simulink model "system_model"  (R2024a)
settings: Solver=VariableStepAuto  StartTime=0.0  StopTime=100000.0  MaxStep=1  RelTol=1e-9
values from neighbouring files (symbols this model uses):
  a_leader = 500*10^3 + earth_radi    (= 6871000)    [main.m]    (also in main_2.m)
  B_f_max = (C_d*A_f_max)/m_f    (= 0.78)    [main_2.m]
  B_f_min = (C_d*A_f_min)/m_f    (= 0.13)    [main_2.m]
  B_l_max = (C_d*A_l_max)/m_l    (= 0.78)    [main_2.m]
  B_l_min = (C_d*A_l_min)/m_l    (= 0.13)    [main_2.m]
  earth_radi = 6371*10^3    (= 6371000)    [main.m]    (also in main_2.m)
  J = eye(3)    [attitude.m]    (also in state_func.m = 43943563035.8; state_func_test.m = J_2 * R_E^2)
  J_2 = 1.08263 * 10^(-3)    (= 0.00108263)    [main.m]    (also in main_2.m; state_func.m)
  Kd = 5    [attitude.m]
  Kp = 5    [attitude.m]
  m_f = 1    [main.m]    (also in main_2.m = 2)
  m_l = 1    [main.m]    (also in main_2.m = 2)
  mu = 13/ 26.98    (= 0.481838398814)    [drag_coefficent_ruff_estimation.m]    (also in main.m = 6.67e-11; main_2.m = 398589196000000; state_func.m = 398589196000000; untitled5.m)
  q_0 = q_0 /norm(q_0)    [attitude.m]
  rho_leader = mean_rho_500km    (= 7.3e-13)    [main_2.m]
  w_0 = [1; 2; 1]    [attitude.m]
  x = theta_vec    [drag_coefficent_ruff_estimation.m]    (also in main.m = [d_a; d_lambda; d_e_x; d_e_y; d_i_x; d_i_y; d_Ballistic]; main_2.m = [d_a; d_lambda; d_e_x; d_e_y; d_i_x; d_i_y])
  x_f_prop = [a_follower; m_follower; e_follower; omega_follower; Omega_follower; i_follower]    [main_2.m]
  x_l_prop = [a_leader; m_leader; e_leader; omega_leader; Omega_leader; i_leader]    [main_2.m]
libraries: mpclib x1, slpidlib x1
(part 1 of 2)
settings Model: Creator=andrefan  LastModifiedBy=andre
settings DataIOCC: FinalStateName=system_modelSimState  InitialState=system_modelSimState  SaveFinalState=on  SaveOperatingPoint=on
settings RTWCC: GPUComputeCapability=3.5

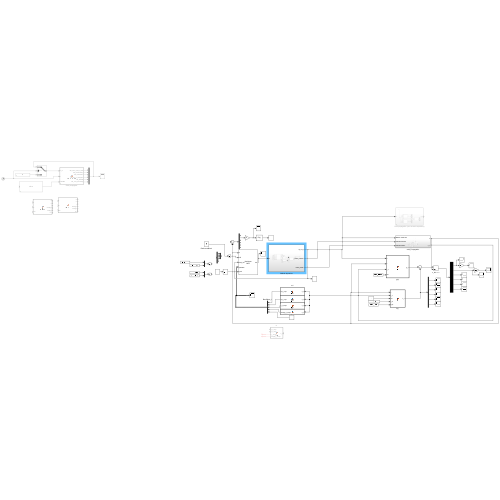
[thumbnail: Simulink's stored preview of the top-level diagram]
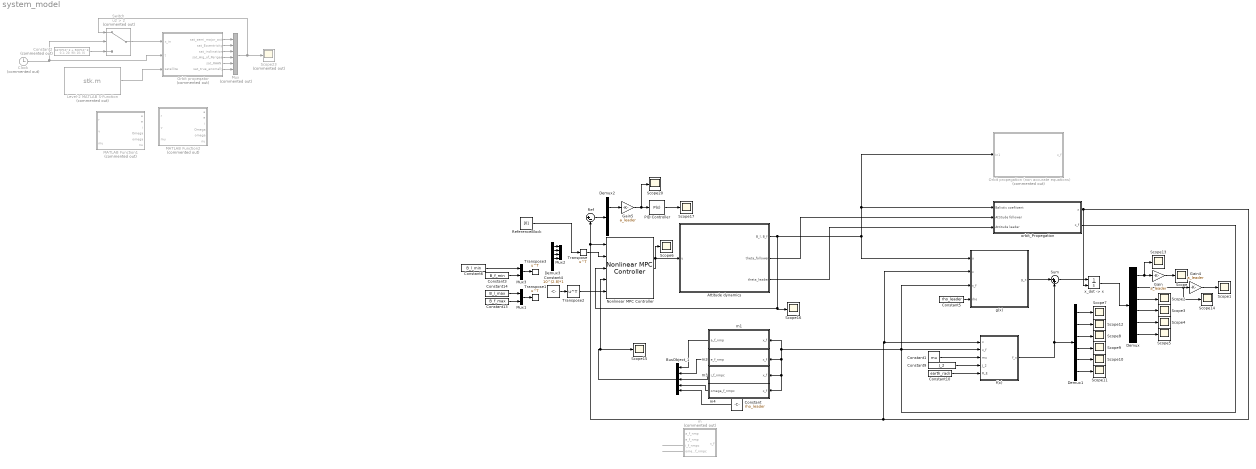
== system system_model ==
  Attitude dynamics : Subsystem
  BusObject_1 : BusCreator  Inputs=5  OutDataTypeStr=Bus: BusObject  NonVirtualBus=on
      settings: InheritFromInputs=off
  Clock : Clock  Commented=on
  Constant : Constant  Value=rho_leader
  Constant1 : Constant  Value=mu
  Constant10 : Constant  Value=earth_radi
  Constant13 : Constant  Value=B_f_max
  Constant14 : Constant  Value=B_l_max
  Constant2 : Constant  Commented=on  Value=|
      | [6370*10^3 + 500*10^3; 0.1;
      | 20; 90;
      | 10;
      | 0]
  Constant3 : Constant  Value=B_f_min
  Constant4 : Constant  Value=10^(2.8)*1
  Constant5 : Constant  Value=rho_leader
  Constant6 : Constant  Value=B_l_min
  Constant9 : Constant  Value=J_2
  Demux{,1..3} (4 alike) : Demux  Outputs=6
  Gain : Gain  Gain=a_leader
  Gain4 : Gain  Gain=a_leader
  Gain5 : Gain  Gain=a_leader
  Level-2 MATLAB S-Function : M-S-Function  Commented=on  FunctionName=stk.m
  MATLAB Function1 : MATLAB Function  Commented=on  TreatAsAtomicUnit=on
  MATLAB Function2 : MATLAB Function  Commented=on  TreatAsAtomicUnit=on
  Mux : Mux  Commented=on  Inputs=6
  Mux1 : Mux  Inputs=2
  Mux2 : Mux
  Mux3 : Mux  Inputs=2
  Nonlinear MPC Controller : mpclib/Nonlinear MPC Controller  nlmpcobj=nlobj  UseObjectTs=on  TsControl=20  UseMEX=off  md_enabled=off  mvtarget_enabled=off  param_enabled=on  cost_enabled=off  mvseq_enabled=off  stateseq_enabled=off  ovseq_enabled=off  slack_enabled=off  status_enabled=off  ov_min=off  ov_max=off  mv_min=off  mv_max=off  mvrate_min=off  mvrate_max=off  state_min=off  state_max=off  ov_weight=on  mv_weight=off  mvrate_weight=off  ecr_weight=off  nlp_initialize=off
  Orbit propegation (non accurate equations) : Subsystem  Commented=on
  Orbit propegator : MATLAB Function  Commented=on  TreatAsAtomicUnit=on
  PID Controller : slpidlib/PID Controller  Controller=P  Form=Parallel  TimeDomain=Continuous-time  UseExternalTs=off  SampleTime=-1  IntegratorMethod=Forward Euler  FilterMethod=Forward Euler  ControllerParametersSource=internal  P=500  I=0.002  UseKiTs=off  D=0  UseExternalDerivativeSource=off  N=100  UseFilter=on  TunerSelectOption=Transfer Function Based (PID Tuner App)  InitialConditionSource=internal  InitialConditionForIntegrator=0  InitialConditionForFilter=0  DifferentiatorICPrevScaledInput=0  ExternalReset=none  TrackingMode=off  Kt=1  LimitOutput=off  SatLimitsSource=internal  UpperSaturationLimit=inf  LowerSaturationLimit=-inf  LinearizeAsGain=on  AntiWindupMode=none  Kb=1  LimitIntegrator=off  UpperIntegratorSaturationLimit=inf  LowerIntegratorSaturationLimit=-inf  POutMin=[]  POutMax=[]  IOutMin=[]  IOutMax=[]  DOutMin=[]  DOutMax=[]  NOutMin=[]  NOutMax=[]  SumOutMin=[]  SumOutMax=[]  SaturationOutMin=[]  SaturationOutMax=[]  PParamMin=[]  PParamMax=[]  IParamMin=[]  IParamMax=[]  DParamMin=[]  DParamMax=[]  NParamMin=[]  NParamMax=[]  KbParamMin=[]  KbParamMax=[]  KtParamMin=[]  KtParamMax=[]  KbOutMin=[]  KbOutMax=[]  KtOutMin=[]  KtOutMax=[]  IntegratorOutMin=[]  IntegratorOutMax=[]  FilterOutMin=[]  FilterOutMax=[]  SumI1OutMin=[]  SumI1OutMax=[]  SumI2OutMin=[]  SumI2OutMax=[]  SumI3OutMin=[]  SumI3OutMax=[]  SumI4OutMin=[]  SumI4OutMax=[]  SumDOutMin=[]  SumDOutMax=[]  DifferentiatorOutMin=[]  DifferentiatorOutMax=[]  FilterDiffOutCoefMin=[]  FilterDiffOutCoefMax=[]  ReciprocalOutMin=[]  ReciprocalOutMax=[]  SumDenOutMin=[]  SumDenOutMax=[]  SumNumOutMin=[]  SumNumOutMax=[]  DivideOutMin=[]  DivideOutMax=[]  UdiffTsProdOutMin=[]  UdiffTsProdOutMax=[]  NTsProdOutMin=[]  NTsProdOutMax=[]  UintegralTsProdOutMin=[]  UintegralTsProdOutMax=[]  UngainTsProdOutMin=[]  UngainTsProdOutMax=[]  ClampingZeroOutDataTypeStr=Inherit: Inherit via back propagation  ClampingZeroOutMin=[]  ClampingZeroOutMax=[]  FilterDenConstantOutDataTypeStr=Inherit: Inherit via back propagation  FilterDenConstantOutMin=[]  FilterDenConstantOutMax=[]  PCopyOutDataTypeStr=Inherit: Inherit via back propagation  PCopyOutMin=[]  PCopyOutMax=[]  NCopyOutDataTypeStr=Inherit: Inherit via back propagation  NCopyOutMin=[]  NCopyOutMax=[]  IntegratorContinuousStateAttributes=''  IntegratorStateMustResolveToSignalObject=off  IntegratorRTWStateStorageClass=Auto  FilterContinuousStateAttributes=''  FilterStateMustResolveToSignalObject=off  FilterRTWStateStorageClass=Auto  ParallelPVariant=InternalParameters  IdealPVariant=Disabled  IVariant=Disabled  DVariant=Disabled  IntegratorVariant=Disabled  SatVariant=Disabled  AWVariant=Disabled  PCopyVariant=Disabled  TRVariant=Disabled  FdbkBlocksVariant=Forward  IdealPFdbkVariant=Disabled  SatFdbkVariant=Disabled  DerivativeFilterVariant=Disabled  NVariant=Disabled  NCopyVariant=Disabled_SignalSpec  FilterICVariant=Disabled  IntegratorICVariant=Disabled  ExternalResetVariant=Disabled  TRSumVariant=Passthrough  SumFdbkVariant=Disabled  SumVariant=Passthrough_P  TsampFilterVariant=InternalTs  TsampNgainVariant=Passthrough  TsampIntegralVariant=Disabled_SignalSpec  ExternalSaturationOutDataTypeStr=Inherit: Same as second input  DerivativeSourceVariant=Disabled
  Ref : Sum  Inputs=|+-
  ReferenceBlock : Constant  Value=[0]
  Scope{,1..17,20} (19 alike) : Scope
  Scope23 : Scope  Commented=on
  Sum : Sum  Inputs=|++
  Switch : Switch  Commented=on  Criteria=u2 > Threshold  Threshold=2  SaturateOnIntegerOverflow=off  InputSameDT=off
  Transpose{,1..3} (4 alike) : Math  Operator=transpose
  f(x) : MATLAB Function  TreatAsAtomicUnit=on
  g(x) : MATLAB Function  TreatAsAtomicUnit=on
  m : MATLAB Function  Commented=on  TreatAsAtomicUnit=on
  m1 : MATLAB Function  TreatAsAtomicUnit=on
  m2 : MATLAB Function  TreatAsAtomicUnit=on
  m3 : MATLAB Function  TreatAsAtomicUnit=on
  m4 : MATLAB Function  TreatAsAtomicUnit=on
  orbit_Propegation : Subsystem
  "x_dot -> x" : Integrator  InitialConditionSource=external  InitialCondition=x
  wires:
  g(x)/1(g_x) -> Sum/1
  Sum/1 -> "x_dot -> x"/1
  "x_dot -> x"/1 -> Demux/1
  f(x)/1(f_x) -> Demux1/1, Sum/2
  Constant1/1 -> f(x)/3(mu)
  Constant5/1 -> g(x)/4(rho)
  Constant9/1 -> f(x)/4(J_2)
  Constant10/1 -> f(x)/5(R_E)
  Demux/3 -> Scope2/1
  Demux/2 -> Scope14/1, Gain4/1
  Demux/1 -> Scope13/1, Gain/1
  Demux/5 -> Scope4/1
  Demux/6 -> Scope5/1
  Demux/4 -> Scope3/1
  Gain/1 -> Scope/1
  Demux1/2 -> Scope12/1
  Gain4/1 -> Scope1/1
  Ref/1 -> Demux2/1
  PID Controller/1 -> Scope17/1
  Demux2/2 -> Gain5/1
  Gain5/1 -> PID Controller/1, Scope20/1
  Attitude dynamics/1("B_l, B_f") -> Scope16/1, Nonlinear MPC Controller/3, g(x)/1(u), Orbit propegation (non accurate equations)/1(In1), orbit_Propegation/1(Balistic coefiicent)
  Clock/1 -> Orbit propegator/2(t), Switch/2
  Constant2/1 -> Switch/3
  Switch/1 -> Orbit propegator/1(x_in)
  Orbit propegator/1(sat_semi_major_axis) -> Mux/1
  Orbit propegator/2(sat_Eccentricity) -> Mux/2
  Orbit propegator/3(sat_inclination) -> Mux/3
  Orbit propegator/4(sat_Arg_of_Perigee) -> Mux/4
  Orbit propegator/5(sat_RAAN) -> Mux/5
  Orbit propegator/6(sat_true_anomally) -> Mux/6
  Mux/1 -> Scope23/1, Switch/1
  Level-2 MATLAB S-Function/1 -> Orbit propegator/3(satellite)
  Attitude dynamics/3(theta_leader) -> orbit_Propegation/3(Attitude leader)
  Attitude dynamics/2(theta_follower) -> orbit_Propegation/2(Attitude follower)
  Nonlinear MPC Controller/1 -> Scope6/1, Attitude dynamics/1(u)
  Constant14/1 -> Mux1/1
  Constant13/1 -> Mux1/2
  Mux1/1 -> Transpose1/1
  Demux1/1 -> Scope7/1
  Demux1/3 -> Scope8/1
  Demux1/4 -> Scope9/1
  Demux1/5 -> Scope10/1
  Demux1/6 -> Scope11/1
  orbit_Propegation/2(x_f) -> m4/1(x_f), m3/1(x_f), m2/1(x_f), m1/1(x_f), f(x)/2(x_f), g(x)/3(x_f)
  BusObject_1/1 -> Scope15/1, Nonlinear MPC Controller/4
  ReferenceBlock/1 -> Transpose/1
  Demux3/1 -> Mux2/1
  Demux3/2 -> Mux2/2
  Demux3/3 -> Mux2/3
  Demux3/4 -> Mux2/4
  orbit_Propegation/1(x) -> "x_dot -> x"/2, g(x)/2(x), f(x)/1(x), Ref/2, Nonlinear MPC Controller/1
  Transpose/1 -> Nonlinear MPC Controller/2
  Constant/1 -> BusObject_1/5
  m/4(omega_f_nmpc) -> ?
  m/3(i_f_nmpc) -> ?
  m1/1(a_f_nmp) -> BusObject_1/1
  m2/1(e_f_nmp) -> BusObject_1/2
  m3/1(i_f_nmpc) -> BusObject_1/3
  m4/1(omega_f_nmpc) -> BusObject_1/4
  Constant4/1 -> Transpose2/1
  Transpose2/1 -> Nonlinear MPC Controller/5
  Constant3/1 -> Mux3/2
  Constant6/1 -> Mux3/1
  Mux3/1 -> Transpose3/1

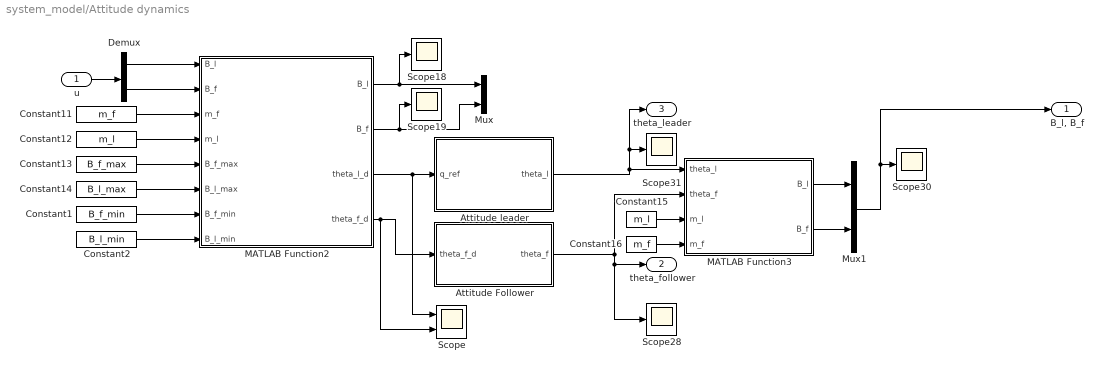
== system system_model/Attitude dynamics ==
  u : Inport
  Attitude Follower : Subsystem
  Attitude leader : Subsystem
  Constant1 : Constant  Value=B_f_min
  Constant11 : Constant  Value=m_f
  Constant12 : Constant  Value=m_l
  Constant13 : Constant  Value=B_f_max
  Constant14 : Constant  Value=B_l_max
  Constant15 : Constant  Value=m_l
  Constant16 : Constant  Value=m_f
  Constant2 : Constant  Value=B_l_min
  Demux : Demux  Outputs=2
  MATLAB Function2 : MATLAB Function  TreatAsAtomicUnit=on
  MATLAB Function3 : MATLAB Function  TreatAsAtomicUnit=on
  Mux : Mux  Inputs=2
  Mux1 : Mux  Inputs=2
  Scope : Scope  NumInputPorts=2
  Scope{18..19,28,30..31} (5 alike) : Scope
  "B_l, B_f" : Outport
  theta_follower : Outport  Port=2
  theta_leader : Outport  Port=3
  wires:
  Constant11/1 -> MATLAB Function2/3(m_f)
  Attitude leader/1(theta_l) -> theta_leader/1, Scope31/1, MATLAB Function3/1(theta_l)
  MATLAB Function2/1(B_l) -> Scope18/1, Mux/1
  Attitude Follower/1(theta_f) -> theta_follower/1, Scope28/1, MATLAB Function3/2(theta_f)
  Demux/2 -> MATLAB Function2/2("B_f ")
  Constant12/1 -> MATLAB Function2/4(m_l)
  MATLAB Function3/1(B_l) -> Mux1/1
  MATLAB Function2/2(B_f) -> Scope19/1, Mux/2
  Constant13/1 -> MATLAB Function2/5(B_f_max)
  Constant14/1 -> MATLAB Function2/6(B_l_max)
  MATLAB Function2/4(theta_f_d) -> Scope/2, Attitude Follower/1(theta_f_d)
  MATLAB Function3/2(B_f) -> Mux1/2
  MATLAB Function2/3(theta_l_d) -> Scope/1, Attitude leader/1(q_ref)
  Constant16/1 -> MATLAB Function3/4(m_f)
  Constant15/1 -> MATLAB Function3/3(m_l)
  Mux1/1 -> "B_l, B_f"/1, Scope30/1
  Constant1/1 -> MATLAB Function2/7(B_f_min)
  Constant2/1 -> MATLAB Function2/8(B_l_min)
  u/1 -> Demux/1
  Demux/1 -> MATLAB Function2/1("B_l ")

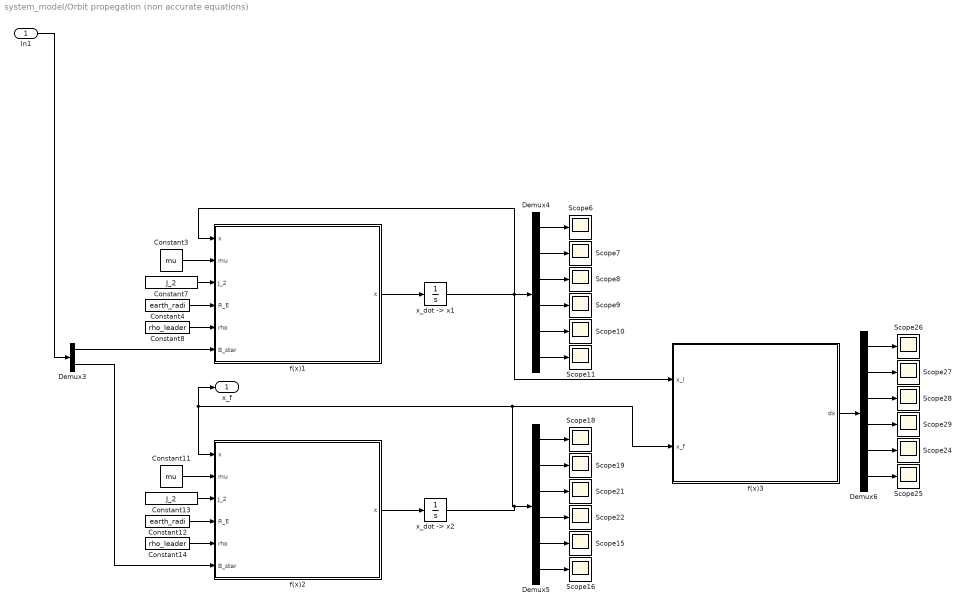
== system system_model/Orbit propegation (non accurate equations) ==
  In1 : Inport
  Constant11 : Constant  Value=mu
  Constant12 : Constant  Value=earth_radi
  Constant13 : Constant  Value=J_2
  Constant14 : Constant  Value=rho_leader
  Constant3 : Constant  Value=mu
  Constant4 : Constant  Value=earth_radi
  Constant7 : Constant  Value=J_2
  Constant8 : Constant  Value=rho_leader
  Demux3 : Demux  Outputs=2
  Demux4 : Demux  Outputs=6
  Demux5 : Demux  Outputs=6
  Demux6 : Demux  Outputs=6
  Scope{6..11,15..16,18..19,21..22,24..29} (18 alike) : Scope
  f(x)1 : MATLAB Function  TreatAsAtomicUnit=on
  f(x)2 : MATLAB Function  TreatAsAtomicUnit=on
  f(x)3 : MATLAB Function  TreatAsAtomicUnit=on
  "x_dot -> x1" : Integrator  InitialCondition=x_l_prop
  "x_dot -> x2" : Integrator  InitialCondition=x_f_prop
  x_f : Outport
  wires:
  Demux4/6 -> Scope11/1
  Constant4/1 -> f(x)1/4(R_E)
  Constant7/1 -> f(x)1/3(J_2)
  Demux3/2 -> f(x)2/6(B_star)
  Demux4/5 -> Scope10/1
  Constant8/1 -> f(x)1/5(rho)
  Demux4/4 -> Scope9/1
  Demux5/4 -> Scope22/1
  Demux5/2 -> Scope19/1
  Demux6/4 -> Scope29/1
  Demux3/1 -> f(x)1/6(B_star)
  Demux4/2 -> Scope7/1
  Constant14/1 -> f(x)2/5(rho)
  Demux4/3 -> Scope8/1
  Constant12/1 -> f(x)2/4(R_E)
  Demux5/5 -> Scope15/1
  Constant11/1 -> f(x)2/2(mu)
  "x_dot -> x1"/1 -> f(x)1/1("x "), Demux4/1, f(x)3/1(x_l)
  Demux5/6 -> Scope16/1
  Demux6/5 -> Scope24/1
  "x_dot -> x2"/1 -> Demux5/1, f(x)3/2(x_f), x_f/1, f(x)2/1("x ")
  Demux6/1 -> Scope26/1
  Demux6/3 -> Scope28/1
  Demux5/1 -> Scope18/1
  f(x)2/1(x) -> "x_dot -> x2"/1
  Constant13/1 -> f(x)2/3(J_2)
  Demux6/2 -> Scope27/1
  Constant3/1 -> f(x)1/2(mu)
  Demux5/3 -> Scope21/1
  Demux6/6 -> Scope25/1
  Demux4/1 -> Scope6/1
  f(x)3/1(dx) -> Demux6/1
  f(x)1/1(x) -> "x_dot -> x1"/1
  In1/1 -> Demux3/1

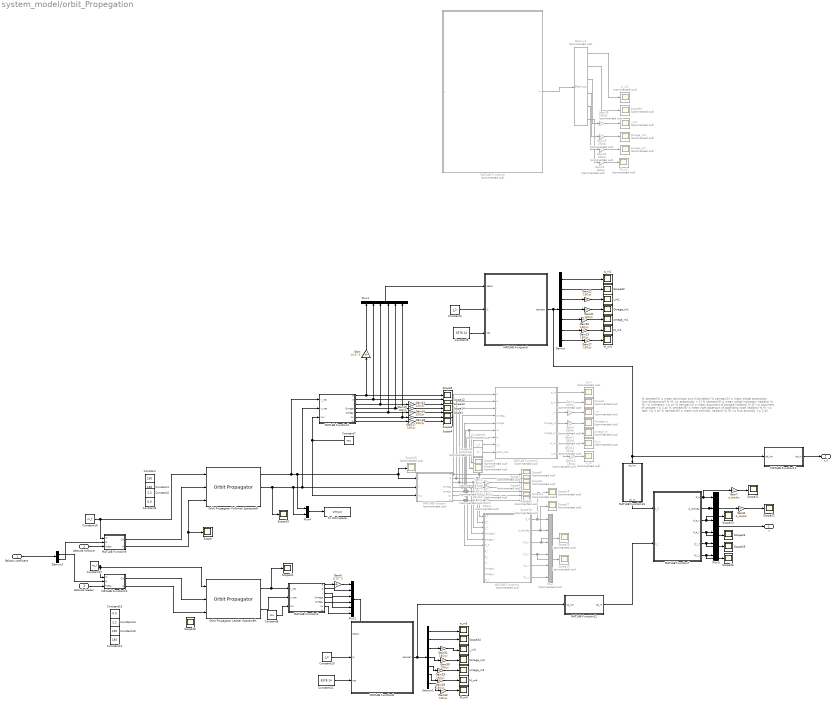
== system system_model/orbit_Propegation ==
  note: % oemean(1) = mean semimajor axis (kilometers)
      | % oemean(2) = mean orbital eccentricity (non-dimensional)
      | % (0 <= eccentricity < 1)
      | % oemean(3) = mean orbital inclination (radians)
      | % (0 <= inclination <= pi)
      | % oemean(4) = mean argument of perigee (radians)
      | % (0 <= argument of perigee <= 2 pi)
      | % oemean(5) = mean right ascension of ascending node (radians)
      | % (0 <= raan <= 2 pi)
      | % oemean(6) = mean true anomaly (radians)
      | % (0 <= true anomaly <= 2 pi)
  Balistic coefiicent : Inport
  Attitude follower : Inport  Port=2
  Attitude leader : Inport  Port=3
  Constant{,1,12..13} (4 alike) : Constant  Value=150
  Constant10 : Constant  Value=J_2
  Constant11 : Constant  Value=6378.14
  Constant14 : Constant  Value=2.2
  Constant15 : Constant  Value=0.0
  Constant16 : Constant  Value=m_f
  Constant17 : Constant  Value=m_l
  Constant2 : Constant  Value=2.2
  Constant3 : Constant  Value=J_2
  Constant4 : Constant  Value=0.0
  Constant5 : Constant  Commented=on  Value=J_2
  Constant6 : Constant  Commented=on  Value=earth_radi
  Constant7 : Constant  Value=mu
  Constant8 : Constant  Value=mu
  Constant9 : Constant  Value=6378.14
  Demux : Demux  Outputs=7
  Demux1 : Demux  Commented=on  Outputs=6
  Demux2 : Demux  Outputs=7
  Demux3 : Demux  Outputs=2
  Gain : Gain  Gain=1/10^3
  Gain{1..5,9..13,23..26} (14 alike) : Gain  Commented=on  Gain=180/pi
  Gain{14..22,27..32} (15 alike) : Gain  Gain=180/pi
  Gain6 : Gain  Gain=1/10^3
  Gain7 : Gain  Gain=a_leader
  Gain8 : Gain  Gain=a_leader
  MATLAB Function : MATLAB Function  Commented=on  TreatAsAtomicUnit=on
  MATLAB Function1 : MATLAB Function  Commented=on  TreatAsAtomicUnit=on
  MATLAB Function10 : MATLAB Function  TreatAsAtomicUnit=on
  MATLAB Function11 : MATLAB Function  TreatAsAtomicUnit=on
  MATLAB Function12 : MATLAB Function  TreatAsAtomicUnit=on
  MATLAB Function13 : MATLAB Function  TreatAsAtomicUnit=on
  MATLAB Function2 : MATLAB Function  TreatAsAtomicUnit=on
  MATLAB Function3 : MATLAB Function  TreatAsAtomicUnit=on
  MATLAB Function4 : MATLAB Function  Commented=on  TreatAsAtomicUnit=on
  MATLAB Function5 : MATLAB Function  TreatAsAtomicUnit=on
  MATLAB Function6 : MATLAB Function  Commented=on  TreatAsAtomicUnit=on
  MATLAB Function7 : MATLAB Function  TreatAsAtomicUnit=on
  MATLAB Function8 : MATLAB Function  TreatAsAtomicUnit=on
  MATLAB Function9 : MATLAB Function  TreatAsAtomicUnit=on
  M_m : Scope  Commented=on
  M_m{1,3..5} (4 alike) : Scope
  M_m2 : Scope  Commented=on
  Mux : Mux  Commented=on  Inputs=6
  Mux1 : Mux  Inputs=6
  Mux2 : Mux  Inputs=6
  Mux3 : Mux  Inputs=6
  Mux4 : Mux  Inputs=2
  Omega_m : Scope  Commented=on
  Omega_m1 : Scope
  Omega_m2 : Scope  Commented=on
  Omega_m3 : Scope
  Orbit Propagator Follower Spacecraft : OrbitPropagator  propagator=Numerical (high precision)  dateOut=off  massSrc=Port  mass=2.0  inclination=20  argPeriapsis=25  trueAnomaly=100  inertialPosition=[3649700.0 3308200.0 -4676600.0]  inertialVelocity=[-2750.8 6666.4 2573.4]  fixedPosition=[-4142689.0 -2676864.7 -4669861.6]  fixedVelocity=[1452.7 -6720.7 2568.1]  gravityModel=Oblate ellipsoid (J2)  customR=3396200  customMu=4.305e13  customJ2=1.0826269e-03  customOmega=4.06125949e-3  outputTransform=on  useDrag=on  useOxygen=off  dragCoeffSrc=Port  dragCoeff=2.3  dragAreaSrc=Port  dragArea=0.6
  Orbit Propagator Leader Spacecraft : OrbitPropagator  propagator=Numerical (high precision)  dateOut=off  massSrc=Port  mass=2.0  inclination=20  argPeriapsis=25  trueAnomaly=100.001  inertialPosition=[3649700.0 3308200.0 -4676600.0]  inertialVelocity=[-2750.8 6666.4 2573.4]  fixedPosition=[-4142689.0 -2676864.7 -4669861.6]  fixedVelocity=[1452.7 -6720.7 2568.1]  gravityModel=Oblate ellipsoid (J2)  customR=3396200  customMu=4.305e13  customJ2=1.0826269e-03  customOmega=4.06125949e-3  useDrag=on  useOxygen=off  dragCoeffSrc=Port  dragCoeff=2.3  dragAreaSrc=Port  dragArea=0.6
  Scope{,1,3..5,12..14,16,21..26,30..32,34} (19 alike) : Scope
  Scope{2,6..11,15,17..20,27..29,33} (16 alike) : Scope  Commented=on
  To Workspace : ToWorkspace  VariableName=simout  SaveFormat=Timeseries  SampleTime=-1
  a_m : Scope  Commented=on
  a_m1 : Scope
  a_m2 : Scope  Commented=on
  a_m3 : Scope
  i_m : Scope  Commented=on
  i_m1 : Scope
  i_m2 : Scope  Commented=on
  i_m3 : Scope
  omega_m : Scope  Commented=on
  omega_m1 : Scope
  omega_m2 : Scope  Commented=on
  omega_m3 : Scope
  u_m : Scope  Commented=on
  x : Outport
  x_f : Outport  Port=2
  wires:
  MATLAB Function/1(a) -> MATLAB Function4/1(a_f), Scope6/1, MATLAB Function1/1(a)
  MATLAB Function4/4(d_e_y) -> Scope29/1, Mux/4
  Gain9/1 -> Scope10/1
  Orbit Propagator Follower Spacecraft/1 -> Mux4/1, MATLAB Function/1(r), Scope15/1, MATLAB Function2/1(r_vec)
  Orbit Propagator Leader Spacecraft/1 -> MATLAB Function3/1(r_vec), Scope31/1
  MATLAB Function4/1(d_a) -> Scope19/1, Mux/1
  MATLAB Function4/6(d_i_y) -> Mux/6
  Gain3/1 -> Scope9/1
  MATLAB Function/3(i) -> MATLAB Function4/3(i_f), Gain1/1, MATLAB Function1/3(i)
  MATLAB Function/7(M) -> MATLAB Function4/6(M_f), Gain10/1, Scope17/1, MATLAB Function1/7(M)
  MATLAB Function4/5(d_i_x) -> Mux/5
  Gain1/1 -> Scope8/1
  Constant7/1 -> MATLAB Function/3(mu), MATLAB Function2/3(mu)
  MATLAB Function/6(nu) -> Gain2/1, Scope20/1, MATLAB Function1/6(nu)
  MATLAB Function4/3(d_e_x) -> Scope28/1, Mux/3
  MATLAB Function4/2(d_lambda) -> Scope27/1, Mux/2
  Gain2/1 -> Scope11/1
  MATLAB Function/2(e) -> MATLAB Function4/2(e_f), Scope7/1, MATLAB Function1/2(e)
  Constant8/1 -> MATLAB Function3/3(mu)
  Gain10/1 -> Scope18/1
  MATLAB Function1/1(a_m) -> a_m/1
  Constant5/1 -> MATLAB Function1/8(J_2)
  Constant6/1 -> MATLAB Function1/9(earth_radi)
  MATLAB Function1/2(e_m) -> Scope2/1
  MATLAB Function1/3(i_m) -> Gain4/1
  MATLAB Function1/4(Omega_m) -> Gain5/1
  MATLAB Function1/5(omega_m) -> Gain11/1
  MATLAB Function1/6(M_m) -> Gain12/1
  Gain4/1 -> i_m/1
  Gain5/1 -> Omega_m/1
  Gain11/1 -> omega_m/1
  Gain12/1 -> M_m/1
  MATLAB Function/5(omega) -> MATLAB Function1/5(omega), MATLAB Function4/5(omega_f), Gain9/1
  MATLAB Function/4(Omega) -> MATLAB Function1/4(Omega), MATLAB Function4/4(Omega_f), Gain3/1
  MATLAB Function1/7(u_m) -> Gain13/1
  Gain13/1 -> u_m/1
  Orbit Propagator Follower Spacecraft/2 -> Mux4/2, MATLAB Function/2(v), MATLAB Function2/2(v_vec), Scope16/1
  MATLAB Function2/7(M) -> Gain18/1
  MATLAB Function2/4(Omega) -> Gain15/1, Mux1/5
  MATLAB Function2/2(e) -> Scope12/1, Mux1/2
  MATLAB Function2/3(i) -> Gain14/1, Mux1/3
  MATLAB Function2/5(omega) -> Gain16/1, Mux1/4
  Gain14/1 -> Scope13/1
  Gain15/1 -> Scope14/1
  Gain16/1 -> Scope1/1
  Gain17/1 -> Scope3/1
  Gain18/1 -> Scope4/1
  Constant3/1 -> MATLAB Function5/2(j2)
  Constant9/1 -> MATLAB Function5/3(req)
  MATLAB Function2/1(a) -> Scope5/1, Gain/1
  MATLAB Function2/6(nu) -> Gain17/1, Mux1/6
  Gain/1 -> Mux1/1
  MATLAB Function5/1(oemean) -> Demux/1, MATLAB Function13/1(ob_km), MATLAB Function11/1(ob_km)
  Demux/6 -> Gain19/1
  Demux/3 -> Gain22/1
  Demux/5 -> Gain20/1
  Demux/2 -> Scope32/1
  Demux/1 -> a_m1/1
  Demux/4 -> Gain21/1
  Gain19/1 -> M_m1/1
  Gain20/1 -> omega_m1/1
  Gain21/1 -> Omega_m1/1
  Gain22/1 -> i_m1/1
  Demux1/2 -> Scope33/1
  Gain23/1 -> M_m2/1
  Gain25/1 -> Omega_m2/1
  Gain24/1 -> omega_m2/1
  Demux1/3 -> Gain26/1
  Gain26/1 -> i_m2/1
  Demux1/5 -> Gain24/1
  Demux1/4 -> Gain25/1
  Demux1/6 -> Gain23/1
  Demux1/1 -> a_m2/1
  MATLAB Function6/1(xn) -> Demux1/1
  Demux/7 -> Gain27/1
  Gain27/1 -> M_m3/1
  Mux1/1 -> MATLAB Function5/1(oeosc)
  Orbit Propagator Leader Spacecraft/2 -> MATLAB Function3/2(v_vec)
  MATLAB Function3/1(a) -> Gain6/1
  MATLAB Function3/2(e) -> Mux2/2
  MATLAB Function3/3(i) -> Mux2/3
  MATLAB Function3/6(nu) -> Mux2/6
  Demux2/7 -> Gain32/1
  Demux2/2 -> Scope34/1
  Demux2/5 -> Gain29/1
  Constant10/1 -> MATLAB Function8/2(j2)
  Gain30/1 -> Omega_m3/1
  Gain29/1 -> omega_m3/1
  Demux2/3 -> Gain31/1
  Gain31/1 -> i_m3/1
  Demux2/4 -> Gain30/1
  Demux2/6 -> Gain28/1
  Constant11/1 -> MATLAB Function8/3(req)
  Gain32/1 -> M_m5/1
  Gain28/1 -> M_m4/1
  Demux2/1 -> a_m3/1
  Mux2/1 -> MATLAB Function8/1(oeosc)
  MATLAB Function8/1(oemean) -> MATLAB Function12/1(ob_km), Demux2/1
  MATLAB Function7/6(d_i_y) -> Scope26/1, Mux3/6
  MATLAB Function7/5(d_i_x) -> Scope25/1, Mux3/5
  MATLAB Function7/4(d_e_y) -> Scope24/1, Mux3/4
  MATLAB Function7/3(d_e_x) -> Scope23/1, Mux3/3
  MATLAB Function7/2(d_lambda) -> Gain8/1, Mux3/2
  MATLAB Function7/1(d_a) -> Gain7/1, Mux3/1
  Mux3/1 -> x/1
  Gain6/1 -> Mux2/1
  MATLAB Function3/5(omega) -> Mux2/4
  MATLAB Function3/4(Omega) -> Mux2/5
  Balistic coefiicent/1 -> Demux3/1
  Attitude follower/1 -> MATLAB Function9/3(theta)
  Attitude leader/1 -> MATLAB Function10/3(theta)
  MATLAB Function10/1(Cd) -> Orbit Propagator Leader Spacecraft/2
  Constant16/1 -> Orbit Propagator Follower Spacecraft/1, MATLAB Function9/1(m)
  Constant17/1 -> MATLAB Function10/1(m), Orbit Propagator Leader Spacecraft/1
  Gain7/1 -> Scope21/1
  Gain8/1 -> Scope22/1
  Demux3/1 -> MATLAB Function10/2(B)
  Demux3/2 -> MATLAB Function9/2(B)
  MATLAB Function10/2(A) -> Orbit Propagator Leader Spacecraft/3
  Mux4/1 -> To Workspace/1
  MATLAB Function11/1(ob_m) -> x_f/1
  MATLAB Function13/1(ob_m) -> MATLAB Function7/1(x_f)
  MATLAB Function12/1(ob_m) -> MATLAB Function7/2(x_l)
  MATLAB Function9/2(A) -> Orbit Propagator Follower Spacecraft/3, Scope/1
  MATLAB Function9/1(Cd) -> Orbit Propagator Follower Spacecraft/2

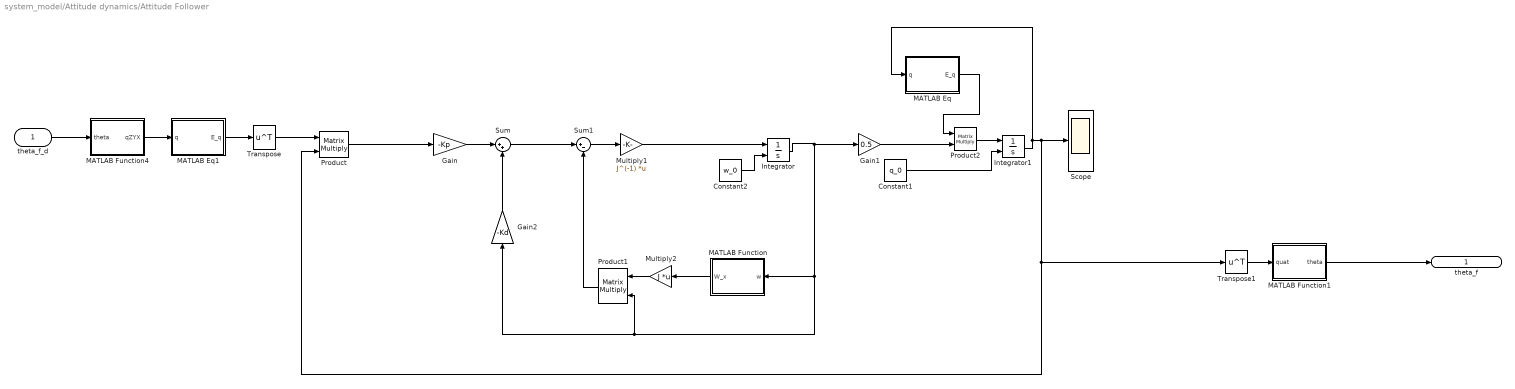
== system system_model/Attitude dynamics/Attitude Follower ==
  theta_f_d : Inport
  Constant1 : Constant  Value=q_0  VectorParams1D=off
  Constant2 : Constant  Value=w_0  VectorParams1D=off
  Gain : Gain  Gain=-Kp
  Gain1 : Gain  Gain=0.5
  Gain2 : Gain  Gain=-Kd
  Integrator : Integrator  InitialConditionSource=external  ContinuousStateAttributes='w'
  Integrator1 : Integrator  InitialConditionSource=external  InitialCondition=[0 0 0 1];  ContinuousStateAttributes='Attitude'
  MATLAB Eq : MATLAB Function  TreatAsAtomicUnit=on
  MATLAB Eq1 : MATLAB Function  TreatAsAtomicUnit=on
  MATLAB Function : MATLAB Function  TreatAsAtomicUnit=on
  MATLAB Function1 : MATLAB Function  TreatAsAtomicUnit=on
  MATLAB Function4 : MATLAB Function  TreatAsAtomicUnit=on
  Multiply1 : Gain  Gain=J^(-1)  Multiplication=Matrix(K*u)
  Multiply2 : Gain  Gain=J  Multiplication=Matrix(K*u)
  Product : Product  Multiplication=Matrix(*)
  Product1 : Product  Multiplication=Matrix(*)
  Product2 : Product  Multiplication=Matrix(*)
  Scope : Scope
  Sum : Sum  Inputs=|++
  Sum1 : Sum  Inputs=|+-
  Transpose : Math  Operator=transpose
  Transpose1 : Math  Operator=transpose
  theta_f : Outport
  wires:
  Sum1/1 -> Multiply1/1
  Product/1 -> Gain/1
  Integrator/1 -> MATLAB Function/1(w), Product1/2, Gain2/1, Gain1/1
  MATLAB Function/1(W_x) -> Multiply2/1
  Product2/1 -> Integrator1/1
  Gain/1 -> Sum/1
  Product1/1 -> Sum1/2
  Sum/1 -> Sum1/1
  Gain1/1 -> Product2/2
  Multiply2/1 -> Product1/1
  Multiply1/1 -> Integrator/1
  MATLAB Eq/1(E_q) -> Product2/1
  Gain2/1 -> Sum/2
  Constant1/1 -> Integrator1/2
  Constant2/1 -> Integrator/2
  MATLAB Eq1/1(E_q) -> Transpose/1
  Transpose/1 -> Product/1
  theta_f_d/1 -> MATLAB Function4/1(theta)
  MATLAB Function4/1(qZYX) -> MATLAB Eq1/1(q)
  Integrator1/1 -> MATLAB Eq/1(q), Product/2, Transpose1/1, Scope/1
  Transpose1/1 -> MATLAB Function1/1(quat)
  MATLAB Function1/1(theta) -> theta_f/1

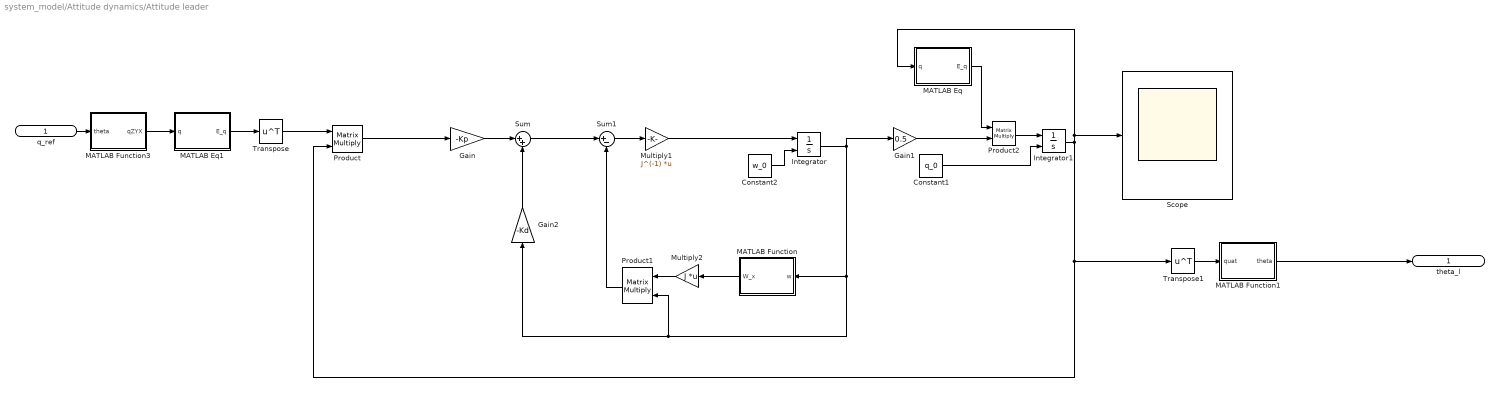
== system system_model/Attitude dynamics/Attitude leader ==
  q_ref : Inport
  Constant1 : Constant  Value=q_0  VectorParams1D=off
  Constant2 : Constant  Value=w_0  VectorParams1D=off
  Gain : Gain  Gain=-Kp
  Gain1 : Gain  Gain=0.5
  Gain2 : Gain  Gain=-Kd
  Integrator : Integrator  InitialConditionSource=external
  Integrator1 : Integrator  InitialConditionSource=external  InitialCondition=[0 0 0 1];
  MATLAB Eq : MATLAB Function  TreatAsAtomicUnit=on
  MATLAB Eq1 : MATLAB Function  TreatAsAtomicUnit=on
  MATLAB Function : MATLAB Function  TreatAsAtomicUnit=on
  MATLAB Function1 : MATLAB Function  TreatAsAtomicUnit=on
  MATLAB Function3 : MATLAB Function  TreatAsAtomicUnit=on
  Multiply1 : Gain  Gain=J^(-1)  Multiplication=Matrix(K*u)
  Multiply2 : Gain  Gain=J  Multiplication=Matrix(K*u)
  Product : Product  Multiplication=Matrix(*)
  Product1 : Product  Multiplication=Matrix(*)
  Product2 : Product  Multiplication=Matrix(*)
  Scope : Scope
  Sum : Sum  Inputs=|++
  Sum1 : Sum  Inputs=|+-
  Transpose : Math  Operator=transpose
  Transpose1 : Math  Operator=transpose
  theta_l : Outport
  wires:
  Sum1/1 -> Multiply1/1
  Product/1 -> Gain/1
  Integrator/1 -> Gain1/1, MATLAB Function/1(w), Gain2/1, Product1/2
  MATLAB Function/1(W_x) -> Multiply2/1
  Product2/1 -> Integrator1/1
  Gain/1 -> Sum/1
  Product1/1 -> Sum1/2
  Sum/1 -> Sum1/1
  Gain1/1 -> Product2/2
  Multiply2/1 -> Product1/1
  Multiply1/1 -> Integrator/1
  Transpose/1 -> Product/1
  MATLAB Eq/1(E_q) -> Product2/1
  Gain2/1 -> Sum/2
  Constant1/1 -> Integrator1/2
  Constant2/1 -> Integrator/2
  Integrator1/1 -> Transpose1/1, Product/2, MATLAB Eq/1(q), Scope/1
  MATLAB Eq1/1(E_q) -> Transpose/1
  q_ref/1 -> MATLAB Function3/1(theta)
  MATLAB Function3/1(qZYX) -> MATLAB Eq1/1(q)
  Transpose1/1 -> MATLAB Function1/1(quat)
  MATLAB Function1/1(theta) -> theta_l/1

== matlab function system_model/Attitude dynamics/Attitude leader/MATLAB Function ==
  data: w input; W_x output
function W_x = Wx(w)
    
      W_x = [0      -w(7-4)   w(6-4);
            w(7-4)     0      -w(5-4);
           -w(6-4)   w(5-4)    0];

== matlab function system_model/Attitude dynamics/Attitude Follower/MATLAB Eq ==
  data: q input; E_q output
function E_q = Eq(q)
      E_q = [q(4)  -q(3)   q(2);
             q(3)   q(4)  -q(1);
            -q(2)   q(1)   q(4);
            -q(1)  -q(2)  -q(3)];

== matlab function system_model/Attitude dynamics/Attitude Follower/MATLAB Eq1 ==
  data: q input; E_q output
function E_q = Eq(q)
      E_q = [q(4)  -q(3)   q(2);
             q(3)   q(4)  -q(1);
            -q(2)   q(1)   q(4);
            -q(1)  -q(2)  -q(3)];

== matlab function system_model/Attitude dynamics/Attitude Follower/MATLAB Function ==
  data: w input; W_x output
function W_x = Wx(w)
    
      W_x = [0      -w(7-4)   w(6-4);
            w(7-4)     0      -w(5-4);
           -w(6-4)   w(5-4)    0];

== matlab function system_model/Attitude dynamics/Attitude leader/MATLAB Function1 ==
  data: quat input; theta output
function theta = QToTheta(quat)
eul = quat2eul( quat );
theta = eul(2);

== matlab function system_model/Attitude dynamics/Attitude Follower/MATLAB Function4 ==
  data: theta input; qZYX output
function qZYX = thetaToQ(theta)
eul = [0 theta 0];
qZYX = eul2quat(eul);

== matlab function system_model/Attitude dynamics/Attitude leader/MATLAB Function3 ==
  data: theta input; qZYX output
function qZYX = thetaToQ(theta)
eul = [0 theta 0];
qZYX = eul2quat(eul);

== matlab function system_model/Attitude dynamics/Attitude Follower/MATLAB Function1 ==
  data: quat input; theta output
function theta = QToTheta(quat)
eul = quat2eul( quat );
theta = eul(2);

== matlab function system_model/Attitude dynamics/MATLAB Function3 ==
  data: B_l output; theta_l input; B_f output; theta_f input; m_l input; m_f input
function [B_l, B_f] = theta_to_ballistic(theta_l, theta_f, m_l, m_f)
%DRAGTOATTITUDE Summary of this function goes here
%   Detailed explanation goes here

    
    A_Cd_l = A_Cd(theta_l);
    A_Cd_f = A_Cd(theta_f);
    
    B_l = A_Cd_l/m_l;
    B_f = A_Cd_f/m_f;

end


% Remember that this function must be updated for different Cd and A
function y = A_Cd(x)
    %y = 40.01*x^4  -411.74*x^3 + 327.3*x^2 + 1173.96*x^1 + 261.12; cm^2
    y = 0.004*x^4 -0.0412 *x^3 + 0.0327*x^2 + 0.1174 *x + 0.0261;   %m^2
end

== matlab function system_model/MATLAB Function2 ==
  data: r input; a output; v input; mu input; e output; i output; Omega output; omega output; nu output
function [a, e, i, Omega, omega, nu] = cart2kep(r, v, mu)
% CART2KEP converts Cartesian coordinates to Keplerian orbital elements
% Input arguments:
% r   - position vector (km)
% v   - velocity vector (km/s)
% mu  - gravitational parameter (km^3/s^2)
% Output arguments:
% a     - semi-major axis (km)
% e     - eccentricity
% i     - inclination (rad)
% Omega - right ascension of the ascending node (rad)
% omega - argument of perigee (rad)
% E     - eccentric anomaly (rad)

h = cross(r,v);
nhat = cross([0 0 1],h);

evec = ((mag(v)^2-mu/mag(r))*r-dot(r,v)*v)/mu;
e = mag(evec);

energy = mag(v)^2/2-mu/mag(r);

if abs(e-1.0)>eps
   a = -mu/(2*energy);
   p = a*(1-e^2);
else
   p = mag(h)^2/mu;
   a = inf;
end

i = acos(h(3)/mag(h));

Omega = acos(n(1)/mag(n));

if n(2)<0
   Omega = 360-Omega;
end

argp = acos(dot(n,evec)/(mag(n)*e));

if e(3)<0
   argp = 360-argp;
end
nu = acos( dot(evec,r) / (e*mag(r)) );

if dot(r,v)<0
   nu = 360 - nu;
end

== matlab function system_model/orbit_Propegation/MATLAB Function3 ==
  data: r_vec input; a output; v_vec input; mu input; e output; i output; Omega output; omega output; nu output; M output
function [a, e, i, Omega, omega, nu, M] = cart2kep(r_vec, v_vec, mu)
% CART2KEP converts Cartesian coordinates to Keplerian orbital elements
% Input arguments:
% r   - position vector (km)
% v   - velocity vector (km/s)
% mu  - gravitational parameter (km^3/s^2)
% Output arguments:
% a     - semi-major axis (km)
% e     - eccentricity
% i     - inclination (rad)
% Omega - right ascension of the ascending node (rad)
% omega - argument of perigee (rad)
% E     - eccentric anomaly (rad)

r = norm(r_vec);
v = norm(v_vec);
v_r = dot(r_vec/r, v_vec);
v_p = sqrt(v^2 - v_r^2);

% Compute specific angular momentum and its magnitude
h_vec = cross(r_vec, v_vec);
h = norm(h_vec);

i = acos(h_vec(3) / h);


K = [0, 0, 1];
N_vec = cross(K, h_vec);
N = norm(N_vec);
if N_vec(2) > 0
    Omega = acos(N_vec(1)/N);
else
    Omega = 2 * pi - acos(N_vec(1)/N);
end



% [section-5]
e_vec = cross(v_vec, h_vec) / mu - r_vec / r;
e = norm(e_vec);

if e_vec(3) >= 0
    omega = acos(dot(N_vec, e_vec) / (N * e));

else
    omega = 2 * pi - acos(dot(N_vec, e_vec) / (N * e));
end

if v_r >= 0
    nu = acos(dot(e_vec, r_vec) / (e * r));

else
    nu = 2*pi - acos(dot(e_vec, r_vec) / (e * r));

end





%a and M are not from the same source as the rest

% Compute semi-major axis and true anomaly
%a = rp/(1-e^2);
a = 1/( (2/norm(r_vec)-(norm(v_vec)^2/mu)) );
 E = atan2(sqrt(1 - e^2) * sin(nu), e + cos(nu));
 E = mod(E, 2 * pi);
 M = E - e * sin(E);

end

== matlab function system_model/orbit_Propegation/MATLAB Function4 ==
  data: a_f input; d_a output; e_f input; i_f input; d_lambda output; d_e_x output; d_e_y output; d_i_x output; d_i_y output; Omega_f input; omega_f input; M_f input; a_l input; e_l input; i_l input; Omega_l input; omega_l input; M_l input
function [d_a, d_lambda, d_e_x, d_e_y, d_i_x, d_i_y] = toRelOribtialElements(a_f, e_f, i_f, Omega_f, omega_f, M_f, a_l, e_l, i_l, Omega_l, omega_l, M_l)

u_l    = omega_l + M_l;
u_f    = omega_f + M_f;

%d_a          = (a_f - a_l) / a_l;
d_a          = (a_f - a_l) / 6786000;
d_lambda     = u_f - u_l + (Omega_f - Omega_l)*cos(i_l);
d_e_x        = e_f*cos(omega_f) - e_l*cos(omega_l);
d_e_y        = e_f*sin(omega_f) - e_l*sin(omega_l);
d_i_x        = i_f - i_l;
d_i_y        = (Omega_f -Omega_l)*sin(i_l);


end

== matlab function system_model/Orbit propegation (non accurate equations)/f(x)1 ==
  data: x input; mu input; J_2 input; R_E input; rho input; B_star input; x output
function x = orbit_prop(x, mu, J_2, R_E, rho, B_star)
    
    a = x(1);
    M = x(2);
    e = x(3);
    omega = x(4);
    Omega = x(5);
    i     = x(6);
    

    % keplerian motion 
    %lambda_dot = mu*a^(-3/2); 
    M_dot_kep = mu*a^(-3/2);
    
    %Drag pertu
    a_dot = (B_star * f(e)*rho*a)/(1-e);
    e_dot = f(e)*rho*B_star;

    %J_2 from: https://sci-hub.se/https://doi.org/10.2514/1.G002409.
    netta       = sqrt(1-e^2);
    gamma       = (3/4)*( J_2 *(R_E)^2 *sqrt(mu))/(a^(7/2)*netta^4);
    M_dot_J     = gamma*netta*(3*cos(i)^2-1);
    omega_dot   = gamma*(5*cos(i)^2-1);
    Omega_dot   = -2*gamma*cos(i);

    
    

    M_dot = M_dot_kep + M_dot_J;
    i_dot = 0;
    

    x = [a_dot; M_dot; e_dot; omega_dot; Omega_dot; i_dot];

end
    

function f = f(e)
    f = 1.61*10^4*e^0.02701 -1.61*10^4;
end

== matlab function system_model/Orbit propegation (non accurate equations)/f(x)2 ==
  data: x input; mu input; J_2 input; R_E input; rho input; B_star input; x output
function x = orbit_prop(x, mu, J_2, R_E, rho, B_star)
    
    a = x(1);
    M = x(2);
    e = x(3);
    omega = x(4);
    Omega = x(5);
    i     = x(6);
    

    % keplerian motion 
    %lambda_dot = mu*a^(-3/2); 
    M_dot_kep = mu*a^(-3/2);
    
    %Drag pertu
    a_dot = (B_star * f(e)*rho*a)/(1-e);
    e_dot = f(e)*rho*B_star;

    %J_2 from: https://sci-hub.se/https://doi.org/10.2514/1.G002409.
    netta       = sqrt(1-e^2);
    gamma       = (3/4)*( J_2 *(R_E)^2 *sqrt(mu))/(a^(7/2)*netta^4);
    M_dot_J     = gamma*netta*(3*cos(i)^2-1);
    omega_dot   = gamma*(5*cos(i)^2-1);
    Omega_dot   = -2*gamma*cos(i);

    
    

    M_dot = M_dot_kep + M_dot_J;
    i_dot = 0;
    

    x = [a_dot; M_dot; e_dot; omega_dot; Omega_dot; i_dot];

end
    

function f = f(e)
    f = 1.61*10^4*e^0.02701 -1.61*10^4;
end

== matlab function system_model/Orbit propegation (non accurate equations)/f(x)3 ==
  data: x_l input; x_f input; dx output
function dx = rel_orb(x_l, x_f)
    
    a_f = x_f(1);
    M_f = x_f(2);
    e_f = x_f(3);
    omega_f = x_f(4);
    Omega_f = x_f(5);
    i_f     = x_f(6);

    a_l = x_l(1);
    M_l = x_l(2);
    e_l = x_l(3);
    omega_l = x_l(4);
    Omega_l = x_l(5);
    i_l     = x_l(6);
    

    u_l         = omega_l + M_l;  
    u_f         = omega_f + M_f;

    d_a          = (a_f - a_l) / a_l;
    d_lambda     = u_f - u_l + (Omega_f - Omega_l)*cos(i_l);
    d_e_x        = e_f*cos(omega_f) - e_l*cos(omega_l);
    d_e_y        = e_f*sin(omega_f) - e_l*sin(omega_l);
    d_i_x        = i_f - i_l;
    d_i_y        = (Omega_f -Omega_l)*sin(i_l);

    
    dx = [d_a; d_lambda; d_e_x; d_e_y; d_i_x; d_i_y];

== matlab function system_model/Orbit propegator ==
  data: x_in input; t input; sat_semi_major_axis output; sat_Eccentricity output; sat_inclination output; sat_Arg_of_Perigee output; sat_RAAN output; sat_true_anomally output; satellite input
function [sat_semi_major_axis, sat_Eccentricity, sat_inclination, sat_Arg_of_Perigee,  sat_RAAN,  sat_true_anomally]= stk_orbitprop(x_in, t, satellite)

    if t < 2
        % x_in = zeros(6,1);
        % x_in(1)=6370*10^3 + 500*10^3;
        % x_in(2)=0.1;
        % x_in(3)=20;
        % x_in(4)= 90;
        % x_in(5)=10;
        % x_in(6)=0;



    end

    sat_semi_major_axis = x_in(1);
    sat_Eccentricity    = x_in(2);
    sat_inclination     = x_in(3);
    sat_Arg_of_Perigee  = x_in(4);
    sat_RAAN            = x_in(5);
    sat_true_anomally   = x_in(6);
   
    %Propegate 
    keplerian.SizeShape.SemiMajorAxis = sat_semi_major_axis;
    keplerian.SizeShape.Eccentricity  = sat_Eccentricity;
    keplerian.Orientation.Inclination = sat_inclination;
    keplerian.Orientation.ArgOfPerigee = sat_Arg_of_Perigee;
    keplerian.Orientation.AscNode.Value     = sat_RAAN;
    keplerian.Location.Value = sat_true_anomally;
    %keplerian.AssignClassical()
    %keplerian.OrbitStateType
    forceModel.Drag.DragModel.Cd=2.2;
    forceModel.Drag.DragModel.AreaMassRatio=0.03;
    %keplerian.AssignClassical('ICRF', 6870000, 0.1, 20, 90, 0, 0);
    satellite.Propagator.InitialState.Representation.Assign(keplerian);
    satellite.Propagator.Propagate();


    %Extract
    root.UnitPreferences.Item('DateFormat').SetCurrentUnit('EpSec');
    satPosDP = satellite.DataProviders.Item('Classical Elements').Group.Item('ICRF').Exec(scenario.StartTime+t,scenario.StartTime+t,t);
    sat_true_anomally = cell2mat(satPosDP.DataSets.GetDataSetByName('True Anomaly').GetValues);
    sat_mean_anomally = cell2mat(satPosDP.DataSets.GetDataSetByName('Mean Anomaly').GetValues);
    sat_semi_major_axis = cell2mat(satPosDP.DataSets.GetDataSetByName('Semi-major Axis').GetValues);
    sat_inclination = cell2mat(satPosDP.DataSets.GetDataSetByName('Inclination').GetValues);
    sat_RAAN = cell2mat(satPosDP.DataSets.GetDataSetByName('RAAN').GetValues);
    sat_Arg_of_Perigee= cell2mat(satPosDP.DataSets.GetDataSetByName('Arg of Perigee').GetValues);
    sat_Eccentricity= cell2mat(satPosDP.DataSets.GetDataSetByName('Eccentricity').GetValues);

     %x = sat_semi_major_axis; sat_Eccentricity; sat_inclination; sat_Arg_of_Perigee;  sat_RAAN;  sat_true_anomally;


end

== matlab function system_model/orbit_Propegation/MATLAB Function1 ==
  data: a input; a_m output; e input; i input; e_m output; i_m output; Omega_m output; omega_m output; M_m output; Omega input; omega input; nu input; M input; J_2 input; earth_radi input; u_m output
function [a_m, e_m, i_m, Omega_m, omega_m, M_m, u_m] = occ2mean_orbital(a, e, i, Omega, omega, nu, M, J_2, earth_radi)

    %% Osculating orbital elements to mean orbital elements
    gamma_2 =  - (J_2/2)* ( (earth_radi/a)^2);
    
    netta = sqrt(1 - e^2); % good
    gamma_2_marked = gamma_2 / (netta^4); % good

    a_div_r = (1 + e*cos(nu)) /netta^2 ; %good

    %shift M and nu to be [-pi,pi]

    %nu = nu -pi;



    a_m = a + a*gamma_2 *( ( 3*cos(i)^2 -1) * ( (a_div_r)^3 - 1/(netta^3) )  ...
        + 3*( 1 - cos(i)^2) * (a_div_r)^3 * cos(2*omega +2*nu) ); % good

    helper_cos_4 = (cos(i)^4) / (1 - 5*cos(i)^2)  ;
    
    de_1 = (gamma_2_marked/8) * e * netta^2 *( 1 - 11*cos(i)^2 - 40* helper_cos_4 ) * cos(2*omega); %ok

    de   = de_1 + (netta^2/2) * ( gamma_2 * ( ( ( 3*cos(i)^2-1) / (netta^6)) * ( e*netta + (e/(1+netta)) + 3*cos(nu)...
        + 3 *e*(cos(nu)^2) + e^2*(cos(nu)^3) )  + 3*( (1-cos(i)^2)/(netta^6) )* (e ...
        + 3*cos(nu) + 3*e*(cos(nu)^2) + e^2*cos(nu)^3 )* cos(2*omega + 2*nu) )...
        - gamma_2_marked*( 1-cos(i)^2)*(3*cos(2*omega+nu) + cos(2*omega + 3*nu) ) ); % good (results at least)


    di = - (e*de_1)/(netta^2*tan(i)) + (gamma_2_marked/2) *cos(i)*sqrt(1-cos(i)^2)*(3*cos(2*omega+2*nu) ...
        + 3*e*cos(2*omega+nu) + e*cos(2*omega+3*nu) ); % ok
    
    %not quite lambda 
    lambda_marked = M + omega + Omega + (gamma_2_marked/8)*netta^3 * (1 - 11*cos(i)^2 - 40*( cos(i^4)/(1- 5 *cos(i)^2) ) ) - ...
        gamma_2_marked/16 *( 2 + e^2 -11*(2+3*e^2)*(cos(i)^2)  ...
        -40*(2+5*e^2)* (cos(i)^4/(1-5*cos(i)^2)) -400*e^2*( (cos(i)^6) / ((1-5*cos(i)^2)^2) ) ) ...
        +gamma_2_marked/4 *( (-6)*(1-5*cos(i)^2) *(nu - M + e*sin(nu) ) ...
        + (3-5*cos(i)^2) *(3*sin(2*omega+2*nu) + 3*e*sin(2*omega+nu) ...
        +e*sin(2*omega+3*nu) ) ) ...
        - gamma_2_marked/8 * e^2 *cos(i)*( 11 + 80 * ( (cos(i)^2)/(1-5*cos(i)^2) ) + 200*( (cos(i)^4)/(1-5*cos(i)^2)^2 ) ) ... %changed plus to minus at start of line
        -gamma_2_marked/2 * cos(i)*(6* ( nu - M + e*sin(nu) ) ...
        -3*sin(2*omega+2*nu) -3*e*sin(2*omega+nu) - e*sin(2*omega+3*nu));

    e_dM = (gamma_2_marked/8) * e * netta^3 * (1 - 11*cos(i)^2 -40* helper_cos_4) ...
        -(gamma_2_marked/4) * netta^3 * ( 2 * (3*cos(i)^2 -1)*( (a_div_r*netta)^2 + a_div_r + 1)*sin(nu)  ...
        + 3*(1-cos(i)^2)* ( ( -(a_div_r*netta)^2 - a_div_r + 1 ) * sin(2*omega+nu) ...
        + ( (a_div_r*netta)^2 + a_div_r + (1/3) ) * sin(2*omega + 3*nu) ) );

    dOmega = -gamma_2_marked/8 * e^2 *cos(i)*( 11 + 80 * ( (cos(i)^2)/(1-5*cos(i)^2) ) + 200 *( cos(i)^4 / (1-5*cos(i)^2)^2 ) ) ...
        -gamma_2_marked/2  *cos(i)* ( 6* (nu - M + e*sin(nu)) -3*sin(2*omega+2*nu) ...
        - 3*e*sin(2*omega+nu) -e*sin(2*omega + 3*nu) );

    d_1 = (e + de)*sin(M) + (e_dM)*cos(M);
    d_2 = (e + de)*cos(M) - (e_dM)*sin(M);

    %M_m = atan(d_1/d_2);
    M_m = atan2(-d_2,d_1); % fucked, 100 deg ish phase shift, WHYYYYYYY
    %M_m = atan2(d_2,d_1); % denne stemmer bra med tidligere M
    e_m = sqrt(d_1^2 +d_2^2);

    d_3 = ( sin(i/2) + cos(i/2)*(di/2) ) * sin(Omega) + sin(i/2)*dOmega *cos(Omega);
    d_4 = ( sin(i/2) + cos(i/2)*(di/2) ) * cos(Omega) - sin(i/2)*dOmega *sin(Omega);

    %Omega_m = atan(d_3/d_4);
    Omega_m  = atan2(-d_4,d_3);
    Omega_m  = pi + Omega_m;

    i_m = 2* asin(sqrt(d_3^2 + d_4^2));
    
    %Omega_m = pi/2 - Omega_m; % this almost fixes Omega

    %M_m = pi/2 + M_m; %more correct inital value, but wrong offset from
    M_m = pi + M_m;
    omega_m = lambda_marked - M_m - Omega_m;
    %omega_m = lambda_marked - M - Omega_m;
    
    u_m = lambda_marked - Omega_m;

    %Output correction
   %Omega_m = pi/2 - Omega_m;
   %M_m = pi - M_m;
   %M_m = pi - M_m;
   %omega_m = omega_m;

  
    
end

== matlab function system_model/orbit_Propegation/MATLAB Function2 ==
  data: r_vec input; a output; v_vec input; mu input; e output; i output; Omega output; omega output; nu output; M output
function [a, e, i, Omega, omega, nu, M] = cart2kep(r_vec, v_vec, mu)
% CART2KEP converts Cartesian coordinates to Keplerian orbital elements
% Input arguments:
% r   - position vector (km)
% v   - velocity vector (km/s)
% mu  - gravitational parameter (km^3/s^2)
% Output arguments:
% a     - semi-major axis (km)
% e     - eccentricity
% i     - inclination (rad)
% Omega - right ascension of the ascending node (rad)
% omega - argument of perigee (rad)
% E     - eccentric anomaly (rad)

r = norm(r_vec);
v = norm(v_vec);
v_r = dot(r_vec/r, v_vec);
v_p = sqrt(v^2 - v_r^2);

% Compute specific angular momentum and its magnitude
h_vec = cross(r_vec, v_vec);
h = norm(h_vec);

i = acos(h_vec(3) / h);


K = [0, 0, 1];
N_vec = cross(K, h_vec);
N = norm(N_vec);
if N_vec(2) > 0
    Omega = acos(N_vec(1)/N);
else
    Omega = 2 * pi - acos(N_vec(1)/N);
end



% [section-5]
e_vec = cross(v_vec, h_vec) / mu - r_vec / r;
e = norm(e_vec);

if e_vec(3) >= 0
    omega = acos(dot(N_vec, e_vec) / (N * e));

else
    omega = 2 * pi - acos(dot(N_vec, e_vec) / (N * e));
end

if v_r >= 0
    nu = acos(dot(e_vec, r_vec) / (e * r));

else
    nu = 2*pi - acos(dot(e_vec, r_vec) / (e * r));

end





%a and M are not from the same source as the rest

% Compute semi-major axis and true anomaly
%a = rp/(1-e^2);
a = 1/( (2/norm(r_vec)-(norm(v_vec)^2/mu)) );
 E = atan2(sqrt(1 - e^2) * sin(nu), e + cos(nu));
 E = mod(E, 2 * pi);
 M = E - e * sin(E);

end
